simulink model "SinglePhase_singleStage_BuckBoostInverter"  (R2024b)
settings: Solver=VariableStepAuto  StartTime=0.0  StopTime=1  RelTol=1e-3
libraries: spsVoltageMeasurementLib x10, spsMosfetLib x5, spsSeriesRLCBranchLib x4, spsDiodeLib x3, spsCurrentMeasurementLib x2, spsACVoltageSourceLib x1, simulink x1, spsPVArrayLib x1, spsPowerLib x1, spsTriangleGeneratorLib x1, sps_lib x1
settings Model: Creator=Jatin  LastModifiedBy=Jatin

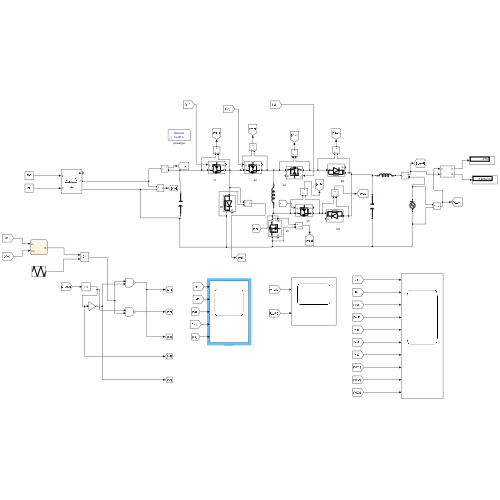
[thumbnail: Simulink's stored preview of the top-level diagram]
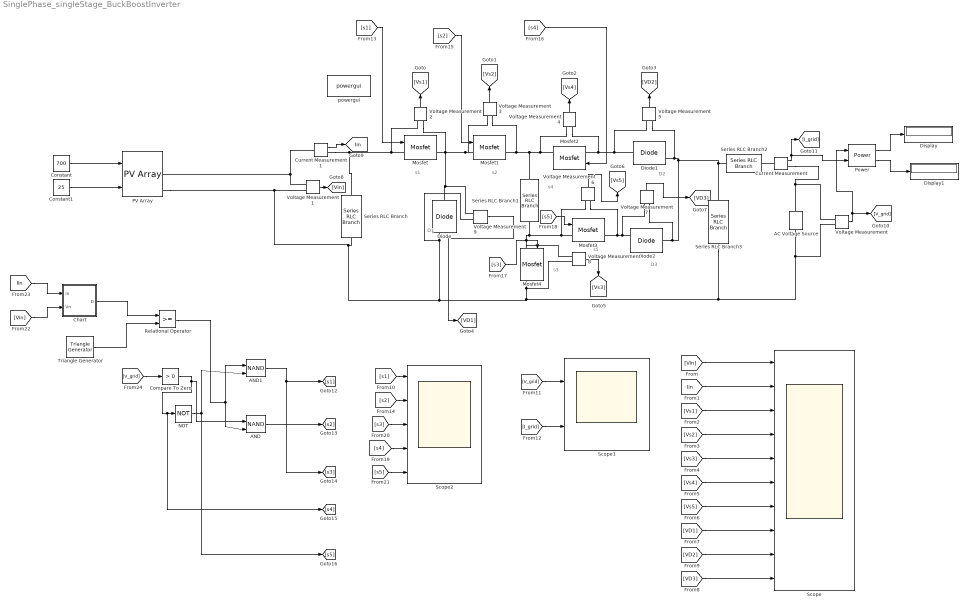
== system SinglePhase_singleStage_BuckBoostInverter ==
  note: D3
  note: D2
  note: D1
  note: s1
  note: s2
  note: s3
  note: s4
  note: s5
  AC Voltage Source : spsACVoltageSourceLib/AC Voltage Source  Amplitude=311  Phase=0  Frequency=50  SampleTime=0  Measurements=None  BusType=swing  Pref=10e3  Qref=0  Qmin=-inf  Qmax=+inf
  AND : Logic  Operator=NAND  IconShape=distinctive  AllPortsSameDT=off  OutDataTypeStr=boolean
  AND1 : Logic  Operator=NAND  IconShape=distinctive  AllPortsSameDT=off  OutDataTypeStr=boolean
  Chart : Stateflow chart  TreatAsAtomicUnit=on
  Compare To Zero : simulink/Logic and Bit Operations/Compare To Zero  relop=>  OutDataTypeStr=boolean
  Constant : Constant  Value=700
  Constant1 : Constant  Value=25
  Current Measurement : spsCurrentMeasurementLib/Current Measurement  PhasorSimulation=off  OutputType=Complex  PSBequivalent=0
  Current Measurement1 : spsCurrentMeasurementLib/Current Measurement  PhasorSimulation=off  OutputType=Complex  PSBequivalent=0
  Diode : spsDiodeLib/Diode  Ron=0.001  Lon=0  Vf=0  IC=0  UseSnubber=0  Rs=500  Cs=250e-9  Measurements=on
  Diode1 : spsDiodeLib/Diode  Ron=0.001  Lon=0  Vf=0  IC=0  UseSnubber=0  Rs=500  Cs=250e-9  Measurements=on
  Diode2 : spsDiodeLib/Diode  Ron=0.001  Lon=0  Vf=0  IC=0  UseSnubber=0  Rs=500  Cs=250e-9  Measurements=on
  Display : Display
  Display1 : Display
  Mosfet{,1..4} (5 alike) : spsMosfetLib/Mosfet  Ron=0.1  Lon=0  Rd=0.01  Vfd=0  IC=0  Rs=1e5  Cs=inf  Measurements=on
  NOT : Logic  Operator=NOT  IconShape=distinctive  AllPortsSameDT=off  OutDataTypeStr=boolean
  PV Array : spsPVArrayLib/PV Array  Npar=40  Nser=10  PlotType=array @ 1000 W/m2 & specified temperatures  S_vec="[ 1000  500  100 ]"  Temp_C_vec="[ 45 25  ]"  ModuleName=User-defined  PlotWhenSelected=off  Pm=87.22  Ncell=60  Voc=22  Isc=5.4  Vm=17.8  Im=4.9  beta_Voc_pc=-0.36099  alpha_Isc_pc=0.102  beta_Voc=-0.079418  alpha_Isc=0.005508  IL=5.4518  I0=1.9938e-10  nI=0.59542  Rsh=66.077  Rs=0.30001  RobustModel=off  RobustCellTemperature=313.3991  BAL=on  Tc=1e-6  Tfilter=5e-5
  Power : spsPowerLib/Power  Freq=60  Vinit=[1, 0]  Iinit=[1, 0]  Ts=0
  Relational Operator : RelationalOperator  OutDataTypeStr=boolean  RndMeth=Simplest  InputSameDT=off
  Scope : Scope  NumInputPorts=10
  Scope1 : Scope  NumInputPorts=2
  Scope2 : Scope  NumInputPorts=5
  Series RLC Branch : spsSeriesRLCBranchLib/Series RLC Branch  LConnTagsString=__new0  RConnTagsString=__new0  BranchType=C  Resistance=1  Inductance=1e-3  SetiL0=off  InitialCurrent=0  Capacitance=10e-6  Setx0=off  InitialVoltage=0  Measurements=None
  Series RLC Branch1 : spsSeriesRLCBranchLib/Series RLC Branch  LConnTagsString=__new0  RConnTagsString=__new0  BranchType=L  Resistance=1  Inductance=10e-6  SetiL0=off  InitialCurrent=0  Capacitance=1e-6  Setx0=off  InitialVoltage=0  Measurements=None
  Series RLC Branch2 : spsSeriesRLCBranchLib/Series RLC Branch  LConnTagsString=__new0  RConnTagsString=__new0  BranchType=L  Resistance=1  Inductance=3.5e-3  SetiL0=off  InitialCurrent=0  Capacitance=1e-6  Setx0=off  InitialVoltage=0  Measurements=None
  Series RLC Branch3 : spsSeriesRLCBranchLib/Series RLC Branch  LConnTagsString=__new0  RConnTagsString=__new0  BranchType=C  Resistance=1  Inductance=1e-3  SetiL0=off  InitialCurrent=0  Capacitance=1e-6  Setx0=off  InitialVoltage=0  Measurements=None
  Triangle Generator : spsTriangleGeneratorLib/Triangle Generator  Freq=1e3  Phase=90  Ts=0
  Voltage Measurement{,1..9} (10 alike) : spsVoltageMeasurementLib/Voltage Measurement  PhasorSimulation=off  OutputType=Complex  PSBequivalent=0
  powergui : sps_lib/powergui  Priority=1  SimulationMode=Discrete  SampleTime=1e-6  frequency=60  Iterations=50  frequencyindice=0  Pbase=100e6  ErrMax=1e-4  UnitsV=kV  UnitsW=MW  buscounter=0  FunctionMessages=off  echomessages=off  EnableUseOfTLC=off  CurrentSourceSwitches=off  DisableSnubberDevices=off  DisableRonSwitches=off  DisableVfSwitches=off  DisplayEquations=off  AutomaticDiscreteSolvers=off  SolverType=Tustin/Backward Euler (TBE)  Interpol=off  ExternalGateDelay=off  methode=off  Ts=100  x0status=blocks  SPID=on  SwTol=0  HookPort=off  NonlinearTolerance=1e-4  nMaxIteration=100  ContinueOnMaxIteration=off  RestoreLinks=warning  ResistiveCurrentMeasurement=off  Frange=[0:2:500]  Ylog=off  Xlog=on  ShowGrid=off  save=off  variable=ZData  structure=0  ZoomFFT=off  StartTime=0.0  cycles=1  DisplayStyle=1  fundamental=60  FreqAxis=off  MaxFrequency=1000  frequencyindicesteady=1  RmsSteady=1  display=off
  tag scope: Iin=global
  wires:
  Constant/1 -> PV Array/1
  Constant1/1 -> PV Array/2
  Voltage Measurement/1 -> [V_grid], Power/1
  Current Measurement/1 -> [I_grid], Power/2
  Voltage Measurement2/1 -> [Vs1]
  Voltage Measurement3/1 -> [Vs2]
  Voltage Measurement4/1 -> [Vs4]
  Voltage Measurement9/1 -> [VD1]
  Voltage Measurement5/1 -> [VD2]
  Voltage Measurement8/1 -> [Vs3]
  Voltage Measurement7/1 -> [VD3]
  Voltage Measurement6/1 -> [Vs5]
  [Vin] -> Scope/1
  [Iin] -> Scope/2
  [Vs1] -> Scope/3
  [Vs2] -> Scope/4
  [Vs3] -> Scope/5
  [Vs4] -> Scope/6
  [Vs5] -> Scope/7
  [VD1] -> Scope/8
  [VD2] -> Scope/9
  [VD3] -> Scope/10
  Power/1 -> Display/1
  Power/2 -> Display1/1
  [V_grid] -> Scope1/1
  [I_grid] -> Scope1/2
  AND/1 -> [s2]
  Compare To Zero/1 -> AND/1, [s4], NOT/1
  NOT/1 -> AND1/2, [s5]
  [s1] -> Mosfet/1
  [s2] -> Mosfet1/1
  [s4] -> Mosfet2/1
  [s5] -> Mosfet3/1
  [s3] -> Mosfet4/1
  [s1] -> Scope2/1
  [s2] -> Scope2/2
  [s4] -> Scope2/4
  [s3] -> Scope2/3
  [s5] -> Scope2/5
  [Vin] -> Chart/2(Vn)
  [Iin] -> Chart/1(In)
  Chart/1(D) -> Relational Operator/1
  Triangle Generator/1 -> Relational Operator/2
  [V_grid] -> Compare To Zero/1
  Relational Operator/1 -> AND/2, AND1/1
  Current Measurement1/1 -> [Iin]
  Voltage Measurement1/1 -> [Vin]
  AND1/1 -> [s3], [s1]
  connections:
  Voltage Measurement2/LConn1 -- Mosfet/LConn1 -- Current Measurement1/RConn1 -- Series RLC Branch/LConn1
  Mosfet1/LConn1 -- Voltage Measurement9/LConn1 -- Diode/LConn1 -- Voltage Measurement2/LConn2 -- Mosfet/RConn1 -- Voltage Measurement3/LConn1
  Mosfet2/RConn1 -- Voltage Measurement3/LConn2 -- Mosfet1/RConn1 -- Series RLC Branch1/LConn1 -- Voltage Measurement4/LConn1
  Diode1/LConn1 -- Voltage Measurement4/LConn2 -- Mosfet2/LConn1 -- Voltage Measurement5/LConn1
  Diode2/RConn1 -- Voltage Measurement7/LConn1 -- Voltage Measurement6/LConn2 -- Mosfet3/RConn1
  Mosfet4/LConn1 -- Voltage Measurement6/LConn1 -- Mosfet3/LConn1 -- Series RLC Branch1/RConn1 -- Voltage Measurement8/LConn1
  Series RLC Branch2/RConn1 -- Voltage Measurement5/LConn2 -- Diode1/RConn1 -- Voltage Measurement7/LConn2 -- Diode2/LConn1 -- Series RLC Branch3/LConn1
  Series RLC Branch3/RConn1 -- AC Voltage Source/LConn1 -- Voltage Measurement/LConn2 -- Voltage Measurement9/LConn2 -- Diode/RConn1 -- Voltage Measurement1/LConn2 -- PV Array/RConn2 -- Series RLC Branch/RConn1 -- Voltage Measurement8/LConn2 -- Mosfet4/RConn1
  Voltage Measurement/LConn1 -- Current Measurement/RConn1 -- AC Voltage Source/RConn1
  Current Measurement1/LConn1 -- Voltage Measurement1/LConn1 -- PV Array/RConn1
  Current Measurement/LConn1 -- Series RLC Branch2/LConn1

== stateflow chart SinglePhase_singleStage_BuckBoostInverter/Chart ==
  state Sense
    Vn,In
  state calculate
    dI=In-Ip
    dV=Vn-Vp
  state J_CheckCurrent
  state J_CheckSlope
    slope_check = In + (dI/dV)*Vn
  state No_change
  state No_change1
  state Increase_D1
  state Decrease_D
  state Increase_D
  state Decrease_D1
  state Return
    Vp = Vn; Ip = In
  (default) -> Sense
  Sense -> calculate
  calculate -> J_CheckCurrent [order 2] : [dV==0]
  calculate -> J_CheckSlope [order 1] : [dV~=0]
  J_CheckCurrent -> No_change1 [order 1] : [dI == 0]
  J_CheckCurrent -> Decrease_D1 [order 2] : [dI>0]{D = D - deltaD}
  J_CheckCurrent -> Increase_D1 [order 3] : [dI<0]{D = D + deltaD}
  J_CheckSlope -> No_change [order 1] : [slope_check == 0]
  J_CheckSlope -> Decrease_D [order 2] : [slope_check > 0]{D = D - deltaD}
  J_CheckSlope -> Increase_D [order 3] : [slope_check < 0]{D = D + deltaD}
  No_change1 -> Return
  No_change -> Return
  Increase_D -> Return
  Increase_D1 -> Return
  Decrease_D -> Return
  Decrease_D1 -> Return
  data: In input; Vn input; Vp local double =0; Ip local double =0; deltaD constant double =0.001; D output =0.5; slope_check local; dV local; dI local
